simulink model "gm_HDLFixedPoint_vs"  (R2024a)
settings: Solver=FixedStepDiscrete  StartTime=0.0  StopTime=stopTime  RelTol=1e-3
undefined symbols (not defined in the file or in its folder): clk, clk_enable, reset_x
libraries: dspsrcs4 x2, simulink x1, vivadosimlib x1
settings Model: Creator=cotti  LastModifiedBy=cotti
settings OptimizationCC: BlockReduction=off  ConditionallyExecuteInputs=off  DefaultParameterBehavior=Inlined  InheritOutputTypeSmallerThanSingle=on
settings DebuggingCC: AlgebraicLoopMsg=error  InheritedTsInSrcMsg=none  SingleTaskRateTransMsg=error  UnconnectedInputMsg=warning  UnconnectedOutputMsg=warning  UnconnectedLineMsg=warning
settings HardwareCC: ProdBitPerPointer=32  ProdBitPerSizeT=32  ProdBitPerPtrDiffT=32  ProdLargestAtomicFloat=None  ProdIntDivRoundTo=Undefined  ProdEndianess=Unspecified  ProdWordSize=32  ProdHWDeviceType=ASIC/FPGA->ASIC/FPGA  TargetBitPerLong=64  TargetBitPerPointer=64  TargetBitPerSizeT=64  TargetBitPerPtrDiffT=64  TargetLongLongMode=on  TargetIntDivRoundTo=Zero  TargetEndianess=LittleEndian  TargetWordSize=64  TargetHWDeviceType=Custom Processor->MATLAB Host Computer  ProdEqTarget=off

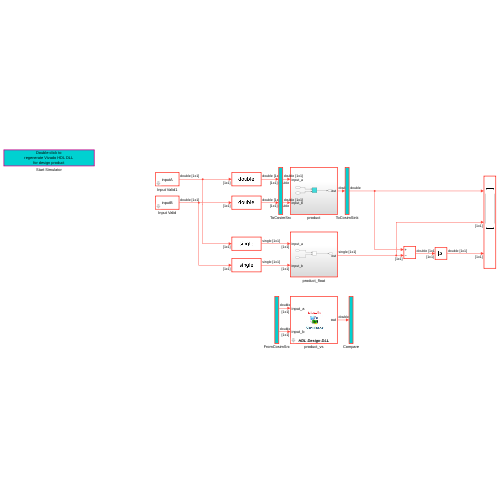
[thumbnail: Simulink's stored preview of the top-level diagram]
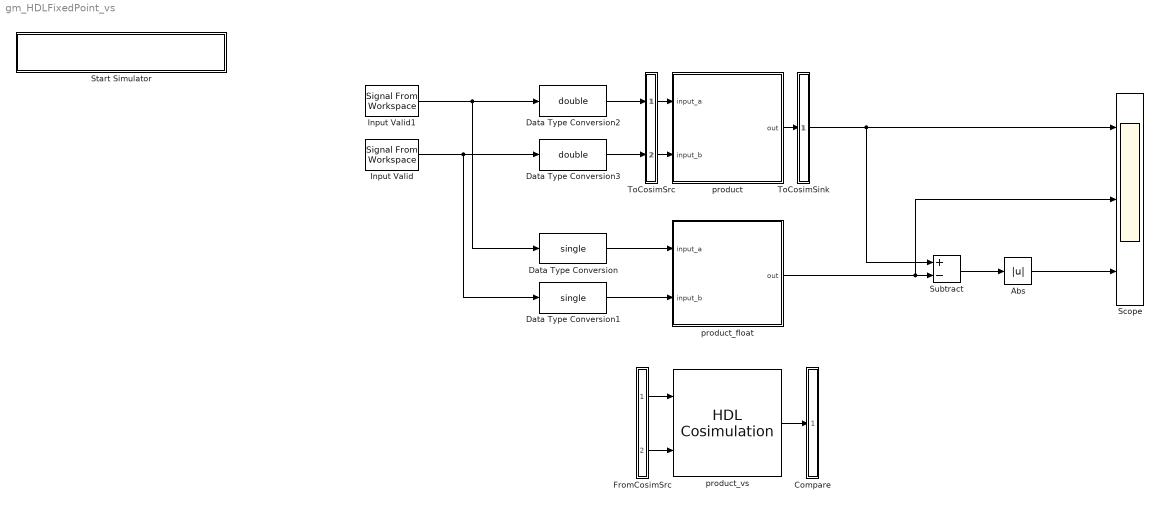
== system gm_HDLFixedPoint_vs ==
  Abs : Abs  SaturateOnIntegerOverflow=off
  Compare : Subsystem
      mask Display: disp('')
  Data Type Conversion : DataTypeConversion  OutDataTypeStr=single  SaturateOnIntegerOverflow=off  RndMeth=Floor
  Data Type Conversion1 : DataTypeConversion  OutDataTypeStr=single  SaturateOnIntegerOverflow=off  RndMeth=Floor
  Data Type Conversion2 : DataTypeConversion  OutDataTypeStr=double  SaturateOnIntegerOverflow=off  RndMeth=Floor
  Data Type Conversion3 : DataTypeConversion  OutDataTypeStr=double  SaturateOnIntegerOverflow=off  RndMeth=Floor
  FromCosimSrc : Subsystem
      mask Display: disp('')
  Input Valid : dspsrcs4/Signal From Workspace  X=inputB  Ts=1  nsamps=1  OutputAfterFinalValue=Setting to zero  ignoreOrWarnInputAndFrameLengths=off  OutputFrames=off
  Input Valid1 : dspsrcs4/Signal From Workspace  X=inputA  Ts=1  nsamps=1  OutputAfterFinalValue=Setting to zero  ignoreOrWarnInputAndFrameLengths=off  OutputFrames=off
  Scope : Scope  NumInputPorts=3
  Start Simulator : Subsystem
      settings: OpenFcn=|
      | cosimDirName = pwd;
      | cd 'hdl_prj/hdlsrc/HDLFixedPoint';
      | [s,r] = system('vivado -mode batch -source gm_HDLFixedPoint_vs.tcl','-echo');
      | cd (cosimDirName);
      | clear cosimDirName;
      | if s
      |    error('Failed to create Vivado HDL design DLL using script gm_HDLFixedPoint_vs.tcl.');
      | end
      mask Display: disp('Double-click to\nregenerate Vivado HDL DLL\nfor design product')
  Subtract : Sum  Inputs=+-
  ToCosimSink : Subsystem
      mask Display: disp('')
  ToCosimSrc : Subsystem
      mask Display: disp('')
  product : Subsystem
  product_float : Subsystem
  product_vs : vivadosimlib/HDL Cosimulation  PortPaths=/product/input_a;/product/input_b;/product/out  PortModes=[1 1 2 ]  PortTimes=[-1 -1 1 ]  PortSigns=[-1 -1 2 ]  PortFracLengths=[0,0,0]  PortWordLengths=[-1,-1,64]  PortHDLWordSizes=[64,64,64]  CommLocal=on  CommSharedMemory=on  CommPortNumber=4449  CommShowInfo=on  ClockPaths=clk;clk_enable;reset_x;  ClockModes=[2 4 3]  ClockTimes=[1e-08 3.7e-08 2.7e-08]  TclPostSimCommand="puts \"done\""  TimingMode=ns  TimingScaleFactor=10  idxCellArray={'UNUSED_VAR'}  CosimBypass=Full Simulation  AllowDirectFeedthrough=on  ProductName=EDA Simulator Link VS  RunAutoTimescale=off  HdlClocks=0  PreRunTime=40  PreRunTimeUnit=ns
  wires:
  Input Valid1/1 -> Data Type Conversion/1, Data Type Conversion2/1
  Input Valid/1 -> Data Type Conversion1/1, Data Type Conversion3/1
  Data Type Conversion/1 -> product_float/1(input_a)
  Data Type Conversion1/1 -> product_float/2(input_b)
  product_float/1(out) -> Subtract/2, Scope/2
  Subtract/1 -> Abs/1
  Abs/1 -> Scope/3
  ToCosimSrc/1(out1) -> product/1(input_a)
  ToCosimSrc/2(out2) -> product/2(input_b)
  product/1(out) -> ToCosimSink/1(in1)
  Data Type Conversion2/1 -> ToCosimSrc/1(in1)
  Data Type Conversion3/1 -> ToCosimSrc/2(in2)
  ToCosimSink/1(out1) -> Scope/1, Subtract/1
  FromCosimSrc/1(out1) -> product_vs/1
  FromCosimSrc/2(out2) -> product_vs/2
  product_vs/1 -> Compare/1(in1)

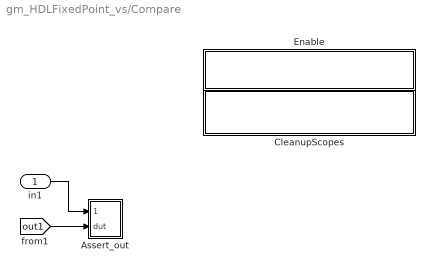
== system gm_HDLFixedPoint_vs/Compare ==
  in1 : Inport
  Assert_out : Subsystem  mask{ToleranceValue=1e-07}
      settings: LibrarySourceBlock=hdlmdlgenlib/AssertRelEq
  CleanupScopes : Subsystem
      settings: OpenFcn=|
      | blkName = gcb; %self block
      | idx = regexp(blkName, '/CleanupScopes$', 'once');
      | blkParent = blkName(1:idx-1);
      | blks=find_system(blkParent, 'LookUnderMasks', 'all','blocktype', 'Scope');
      | for itr = 1:length(blks)
      | 	 hScopeCfg = get_param(blks{itr},'ScopeConfiguration');
      | 	 hScopeCfg.Visible = ~ hScopeCfg.Visible;
      | end
      | drawnow;
      mask Display: fprintf(message('hdlcoder:cosim:vnl_dblclick').getString());
  Enable : Subsystem
      settings: OpenFcn=|
      | blkName = gcb;
      | idx = regexp(blkName, '/Enable$', 'once');
      | blkParent = blkName(1:idx-1);
      | blks=find_system(blkParent, 'LookUnderMasks', 'all','blocktype', 'Assertion');
      | e = get_param(blks{1}, 'Enabled');
      | if strcmp(e, 'on'), f= 'off';, else, f = 'on';, end
      | for ii=1:length(blks), set_param(blks{ii}, 'Enabled', f);, end
      | set_param(gcb, 'MaskDisplay',['fprintf(message(''hdlcoder:cosim:vnl_dblclick_assertions'',','''',upper(e),'''',').getString())']);
      mask Display: fprintf(message('hdlcoder:cosim:vnl_dblclick_assertions','OFF').getString());
  wires:
  [out1] -> Assert_out/2(dut)
  in1/1 -> Assert_out/1(cosim)

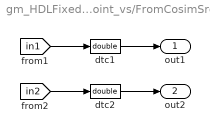
== system gm_HDLFixedPoint_vs/FromCosimSrc ==
  dtc1 : DataTypeConversion  OutDataTypeStr=double
  dtc2 : DataTypeConversion  OutDataTypeStr=double
  out1 : Outport
  out2 : Outport  Port=2
  wires:
  dtc2/1 -> out2/1
  dtc1/1 -> out1/1
  [in2] -> dtc2/1
  [in1] -> dtc1/1

== system gm_HDLFixedPoint_vs/Start Simulator ==

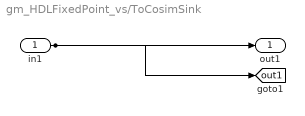
== system gm_HDLFixedPoint_vs/ToCosimSink ==
  in1 : Inport
  out1 : Outport
  tag scope: out1=global
  wires:
  in1/1 -> out1/1, [out1]

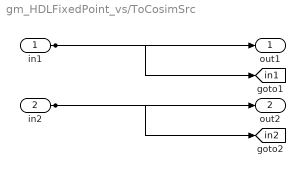
== system gm_HDLFixedPoint_vs/ToCosimSrc ==
  in1 : Inport
  in2 : Inport  Port=2
  out1 : Outport
  out2 : Outport  Port=2
  tag scope: in1=global, in2=global
  wires:
  in1/1 -> out1/1, [in1]
  in2/1 -> out2/1, [in2]

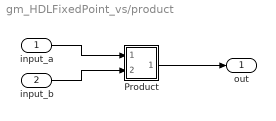
== system gm_HDLFixedPoint_vs/product ==
  input_a : Inport  OutDataTypeStr=double  PortDimensions=1  SampleTime=1
  input_b : Inport  Port=2  OutDataTypeStr=double  PortDimensions=1  SampleTime=1
  Product : Subsystem
      mask Display: disp('NFP\nmul');
  out : Outport  SampleTime=1
  wires:
  Product/1(Out1) -> out/1
  input_b/1 -> Product/2(In2)
  input_a/1 -> Product/1(In1)

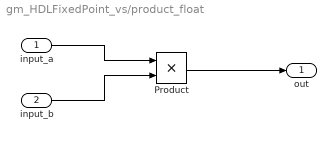
== system gm_HDLFixedPoint_vs/product_float ==
  input_a : Inport
  input_b : Inport  Port=2
  Product : Product
  out : Outport
  wires:
  input_a/1 -> Product/1
  input_b/1 -> Product/2
  Product/1 -> out/1

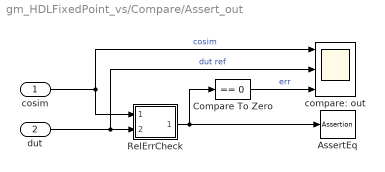
== system gm_HDLFixedPoint_vs/Compare/Assert_out ==
  cosim : Inport
  dut : Inport  Port=2
  AssertEq : Assertion  StopWhenAssertionFail=off
  Compare To Zero : simulink/Logic and Bit Operations/Compare To Zero  relop===  OutDataTypeStr=boolean
  RelErrCheck : Subsystem
  compare: out : Scope  NumInputPorts=3
  wires:
  dut/1 -> compare: out/2, RelErrCheck/2(In2)  "dut ref"
  cosim/1 -> compare: out/1, RelErrCheck/1(In1)  "cosim"
  RelErrCheck/1(Out1) -> AssertEq/1, Compare To Zero/1
  Compare To Zero/1 -> compare: out/3  "err"

== system gm_HDLFixedPoint_vs/Compare/CleanupScopes ==

== system gm_HDLFixedPoint_vs/Compare/Enable ==

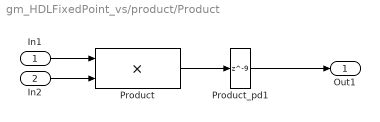
== system gm_HDLFixedPoint_vs/product/Product ==
  In1 : Inport
  In2 : Inport  Port=2
  Product : Product  Inputs=**  OutDataTypeStr=double  SampleTime=1
  Product_pd1 : Delay  DelayLength=9
  Out1 : Outport
  wires:
  Product_pd1/1 -> Out1/1
  Product/1 -> Product_pd1/1
  In2/1 -> Product/2
  In1/1 -> Product/1

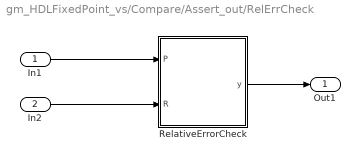
== system gm_HDLFixedPoint_vs/Compare/Assert_out/RelErrCheck ==
  In1 : Inport
  In2 : Inport  Port=2
  "RelativeErrorCheck " : MATLAB Function  TreatAsAtomicUnit=on
  Out1 : Outport  VectorParamsAs1DForOutWhenUnconnected=off
  wires:
  In2/1 -> "RelativeErrorCheck "/2(R)
  In1/1 -> "RelativeErrorCheck "/1(P)
  "RelativeErrorCheck "/1(y) -> Out1/1

== matlab function gm_HDLFixedPoint_vs/Compare/Assert_out/RelErrCheck/RelativeErrorCheck  ==
  data: P input; y output; R input; ToleranceValue parameter double
% Check if the relative error of R with respect to P is below
% ToleranceValue
% P, R are floating-point
function y = relErrCheck(P,R, ToleranceValue)
    tol = ToleranceValue;
    sz = numel(P);
    assert(sz == numel(R), 'Inputs P and R have different sizes.');
    y = false(1, sz);

    for ii=1:sz
        if (isnan(P(ii)) || isnan(R(ii)))
            if (isnan(P(ii)) && isnan(R(ii)))
                y(ii) = true;
            end
        elseif (isinf(P(ii)) || isinf(R(ii)))
            y(ii) = (P(ii) == R(ii));
        elseif (P(ii) == 0)
            y(ii) = (R(ii) == 0);
        else
            absdiff = abs(P(ii) - R(ii));
            relerr = absdiff/abs(P(ii));
            y(ii) = (relerr <= tol);
        end
    end
end
